simulink library "tqd"  (R2021b)
settings: Solver=VariableStepAuto  StartTime=0.0  StopTime=10.0  RelTol=1e-3
undefined symbols (not defined in the file or in its folder): ATQD_AccelLimitInRange_X_rpm, ATQD_AccelLimitInRange_Y_Nm, ATQD_AccelLimitOvrKi_X_Nm, ATQD_AccelLimitOvrKp_X_Nm, ATQD_BOSMapD_X_rpm, ATQD_BOSMapD_Y_pct, ATQD_BOSMapR_X_rpm, ATQD_BOSMapR_Y_pct, ATQD_HVBCurrSmooth_X_A, ATQD_LHMTqMapDLC_X_rpm, ATQD_LHMTqMapDLC_Y_pct, ATQD_LHMTqMapRLC_X_rpm, ATQD_LHMTqMapRLC_Y_pct, ATQD_NormalMapDLC_X_rpm, ATQD_NormalMapDLC_Y_pct, ATQD_NormalTqDecSR_X_rpm, ATQD_NormalTqDecSR_Y_Nm, ATQD_NormalTqIncSR_X_rpm, ATQD_NormalTqIncSR_Y_Nm, ATQD_OPDMapRLC_X_rpm, ATQD_OPDMapRLC_Y_pct, ATQD_RollRegTorReq_X_rpm, ATQD_RollRegTorReq_Y_enum, ATQD_VehSpdLimitInRange_X_rpm, ATQD_VehSpdLimitInRange_Y_Nm, ATQD_VehSpdLimitOvrKi_X_Nm, ATQD_VehSpdLimitOvrKp_X_Nm, EIGHT_INT, ENUM_BRAKEPEDAL_PRESSED, ENUM_BRAKEPEDAL_RELEASED, ENUM_COMBOKEY_DOWN, ENUM_COMBOKEY_M1, ENUM_COMBOKEY_M2, ENUM_COMBOKEY_NONE, ENUM_COMBOKEY_RKNEE, ENUM_COMBOKEY_STOPLV, ENUM_COMBOKEY_UP, ENUM_CP2VKNEEREQ_REQUEST, ENUM_CP2VNLVREQ_LEVEL1, ENUM_CP2VNLVREQ_LEVEL2, ENUM_CP2VNLVREQ_LOWER, ENUM_CP2VNLVREQ_STOPLV, ENUM_CP2VNLVREQ_UPPER, ENUM_CREEPIND_DISABLE, ENUM_CREEPIND_READY, ENUM_CREEPIND_RUNNING, ENUM_CREEPIND_WARNING, ENUM_DRIVELINERELEASE_RELEASE, ENUM_EBSTORQUERWQ_LIMIT, ENUM_EBSTORQUERWQ_TORQUE, ENUM_ECPVCUDRM_CONFORT, ENUM_ECPVCUDRM_ECO, ENUM_ECPVCUDRM_NORMAL, ENUM_ECPVCUDRM_NOTAVAILABLE, ENUM_EMTqModeDrvBrk_Accel, ENUM_EMTqModeDrvBrk_Brake, ENUM_EMTqModeDrvBrk_Coast, ENUM_ETC2ACTDRIVEDIR_BACKWARD, ENUM_ETC2ACTDRIVEDIR_FORWARD, ENUM_ETC2ACTDRIVEDIR_STILL ... (+341)
libraries: simulink x109, hcu_lib x67
(part 6 of 13)

== system tqd/TQD/Input_Convert/Function/Command Limitation ==
  note: Torque Command Lower Limit
  note: Torque Command Upper Limit
  BSCPIn_outputs : Inport
  BSignalConvert_outputs : Inport  Port=2
  VTQD_VehSpdTorLimit_Nm : Inport  Port=3
  VTQD_VehAcclTorLimit_Nm : Inport  Port=4
  Bus Selector : BusSelector  OutputSignals=VTQD_PTAvailMotTq_Nm,VTQD_EM1ReqTorqLimDriv_Nm,VTQD_EM1LimitCtrlDriv_flg,VTQD_TrqLimit_flg,VTQD_EM1ReqTorqLimBrk_Nm,VTQD_EM1LimitCtrlBrk_flg,VTQD_PTAvailGenTq_Nm
  Bus Selector1 : BusSelector  OutputSignals=VDMM_CAN1BUSOFF_flg
  Constant11 : Constant  Value=KTQD_PowerTrainTqLimtAtTargetShaft_Nm
  Constant16 : Constant  Value=KTQD_PowerTrainTqLimtAtTargetShaft_Nm
  Constant21 : Constant  Value=KTQD_PowerTrainTqLimtAtRegen_Nm
  Constant22 : Constant  Value=KTQD_DDMTrqLimitation_Nm
  Constant3 : Constant  Value=KTQD_CAN1BusOffTrqLimit_Nm
  LiuZgSwitch15 : Switch  Criteria=u2 ~= 0  Threshold=0.5
      settings: AttributesFormatString=<%<Criteria>>
  LiuZgSwitch16 : Switch  Criteria=u2 ~= 0  Threshold=0.5
      settings: AttributesFormatString=<%<Criteria>>
  MinMax3 : MinMax  Inputs=6  OutDataTypeStr=single
  MinMax4 : MinMax  Function=max  Inputs=3  OutDataTypeStr=single
  Switch4 : Switch  Criteria=u2 ~= 0
      settings: AttributesFormatString=%<Criteria>
  Switch5 : Switch  Criteria=u2 ~= 0
      settings: AttributesFormatString=%<Criteria>
  VTQD_TqCMDUpLim_Nm : Outport
  VTQD_TqCMDLowLim_Nm : Outport  Port=2
  wires:
  [VTQD_TqCMDLowLim_Nm] -> VTQD_TqCMDLowLim_Nm/1
  Bus Selector1/1 -> [VDMM_CAN1BUSOFF_flg]  "<VDMM_CAN1BUSOFF_flg>"
  BSCPIn_outputs/1 -> Bus Selector1/1
  Bus Selector/1 -> [VTQD_PTAvailMotTq_Nm]  "<VTQD_PTAvailMotTq_Nm>"
  BSignalConvert_outputs/1 -> Bus Selector/1
  VTQD_VehSpdTorLimit_Nm/1 -> [VTQD_VehSpdTorLimit_Nm]
  VTQD_VehAcclTorLimit_Nm/1 -> [VTQD_VehAcclTorLimit_Nm]
  [VTQD_EM1LimitCtrlDriv_flg] -> LiuZgSwitch15/2
  [VDMM_CAN1BUSOFF_flg] -> Switch4/2
  [VTQD_EM1ReqTorqLimDriv_Nm] -> LiuZgSwitch15/1
  Constant3/1 -> Switch4/1
  Constant11/1 -> Switch4/3
  [VTQD_TrqLimit_flg] -> Switch5/2
  Constant16/1 -> Switch5/3
  [VTQD_PTAvailMotTq_Nm] -> LiuZgSwitch15/3
  Constant22/1 -> Switch5/1
  Switch4/1 -> MinMax3/1
  [VTQD_PTAvailMotTq_Nm] -> MinMax3/2
  [VTQD_VehSpdTorLimit_Nm] -> MinMax3/3
  [VTQD_VehAcclTorLimit_Nm] -> MinMax3/4
  LiuZgSwitch15/1 -> MinMax3/5
  Switch5/1 -> MinMax3/6
  Bus Selector/2 -> [VTQD_EM1ReqTorqLimDriv_Nm]  "<VTQD_EM1ReqTorqLimDriv_Nm>"
  Bus Selector/3 -> [VTQD_EM1LimitCtrlDriv_flg]  "<VTQD_EM1LimitCtrlDriv_flg>"
  Bus Selector/4 -> [VTQD_TrqLimit_flg]  "<VTQD_TrqLimit_flg>"
  MinMax3/1 -> [VTQD_TqCMDUpLim_Nm]  "VTQD_TqCMDUpLim_Nm"
  [VTQD_EM1ReqTorqLimBrk_Nm] -> LiuZgSwitch16/1
  [VTQD_PTAvailGenTq_Nm] -> LiuZgSwitch16/3
  [VTQD_EM1LimitCtrlBrk_flg] -> LiuZgSwitch16/2
  Constant21/1 -> MinMax4/1
  LiuZgSwitch16/1 -> MinMax4/2
  [VTQD_PTAvailGenTq_Nm] -> MinMax4/3
  MinMax4/1 -> [VTQD_TqCMDLowLim_Nm]  "VTQD_TqCMDLowLim_Nm"
  Bus Selector/5 -> [VTQD_EM1ReqTorqLimBrk_Nm]  "<VTQD_EM1ReqTorqLimBrk_Nm>"
  Bus Selector/6 -> [VTQD_EM1LimitCtrlBrk_flg]  "<VTQD_EM1LimitCtrlBrk_flg>"
  Bus Selector/7 -> [VTQD_PTAvailGenTq_Nm]  "<VTQD_PTAvailGenTq_Nm>"
  [VTQD_TqCMDUpLim_Nm] -> VTQD_TqCMDUpLim_Nm/1

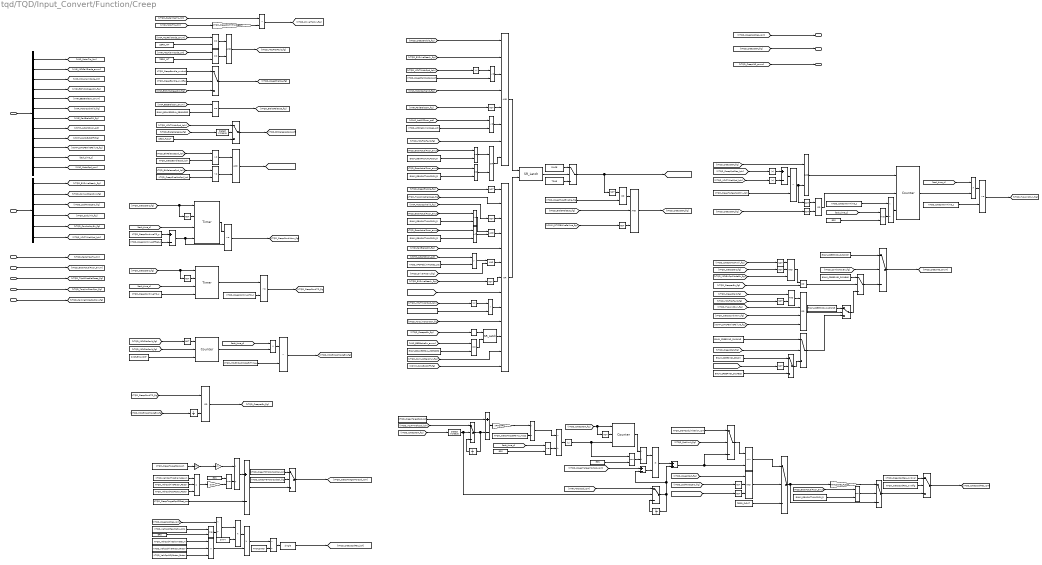
== system tqd/TQD/Input_Convert/Function/Creep ==
  note: TUpA Active Detection
  note: Creep SCP
  note: Creep Enable Judgment
  note: Creep Continue TimeOut
  note: MCU Error Condition
  note: Error Condition Judgment
  note: Unit Convert
  note: CmdSpeedCalculation
  note: Creep Indicate State
  BSCPIn_outputs : Inport
  BSignalConvert_outputs : Inport  Port=2
  VTQD_PedalMapTq_Nm : Inport  Port=3
  VTQD_GearActualPosn_enum : Inport  Port=4
  VTQD_TUpADisableCreep_flg : Inport  Port=5
  VTQD_TorqLimDoorOpn_flg : Inport  Port=6
  VTQD_ParkingProtectAction_flg : Inport  Port=7
  AND{,3,5..8} (6 alike) : Logic  AllPortsSameDT=off  OutDataTypeStr=boolean
  AND1 : Logic  Inputs=3  AllPortsSameDT=off  OutDataTypeStr=boolean
  AND2 : Logic  Inputs=3  AllPortsSameDT=off  OutDataTypeStr=boolean
  AND4 : Logic  Inputs=3  AllPortsSameDT=off  OutDataTypeStr=boolean
  Abs{,1,3..5} (5 alike) : Abs
  Add{,1,3..5} (5 alike) : Sum  Inputs=+-
  Add2 : Sum
  Bus Selector : BusSelector  OutputSignals=VTQD_EVDriveReady_flg,VTQD_ComLostZeroPwr_flg,VTQD_SpdForceZero_flg,VTQD_SpdLimit_flg,VTQD_ComboKeyEn_flg,VTQD_VCUTMVehSpd_kph
  Bus Selector1 : BusSelector  OutputSignals=VINP_MotorTrq_Nm,VINP_MCUFailGrade_enum,VINP_MCUAlarmCode_cnt,VINP_ECPVCUCreepSW_flg,VINP_EBSBrakeSw_enum,VINP_MotorSpdValid_flg,VINP_ParkBrakeSW_flg,VDHP_ActAPSPosn_pct,VDMM_CAN1BUSOFF_flg,VDMM_DTCPBWireFailure_flg,task_time_s,VINP_MotorSpd_rpm
  Constant : Constant  Value=ZERO_FLOAT  OutDataTypeStr=single
  Constant1 : Constant  Value=ENUM_BRAKEPEDAL_PRESSED
  Constant10 : Constant  Value=ENUM_GEARACTUALPOSN_R
  Constant11 : Constant  Value=ENUM_GEARACTUALPOSN_D
  Constant12 : Constant  Value=KTQD_APSPedLim4Creep_pct
  Constant13 : Constant  Value=KTQD_CreepContinueTO_s
  Constant14 : Constant  Value=KTQD_CreepTargetSpd_kph
  Constant15 : Constant  Value=KTQD_VehSpdTireDiameter_m
  Constant16 : Constant  Value=KTQD_VehSpdTireFactor_Factor
  Constant17 : Constant  Value=KTQD_CreepForedEnable_flg
  Constant18 : Constant  Value=KTQD_CreepTargetSpdOffset_rpm
  Constant19 : Constant  Value=KTQD_CreepTGMotorSpdCal_rpm
  Constant2 : Constant  Value=ENUM_GEARACTUALPOSN_R
  Constant20 : Constant  Value=FALSE
  Constant21 : Constant  Value=TRUE
  Constant22 : Constant  Value=ENUM_BRAKEPEDAL_RELEASED
  Constant23 : Constant  Value=ENUM_CREEPIND_DISABLE
  Constant24 : Constant  Value=KTQD_CreepTargetSpd_kph
  Constant25 : Constant  Value=KTQD_CreepTGMotorSpdCal_flg
  Constant26 : Constant  Value=ENUM_GEARACTUALPOSN_R
  Constant27 : Constant  Value=ENUM_GEARACTUALPOSN_D
  Constant28 : Constant  Value=KTQD_CreepTargetRamp_mps2
  Constant29 : Constant  Value=KTQD_CreepSpdReq_ovrdval
  Constant{3,9,31,55..56} (5 alike) : Constant  Value=EPS
  Constant30 : Constant  Value=KTQD_CreepSpdReq_ovrdflg
  Constant32 : Constant  Value=KTQD_CreepWarnTime_s
  Constant33 : Constant  Value=KTQD_CreepTartgerSpdDiv_kph
  Constant34 : Constant  Value=KTQD_VehSpdADJFactor_Factor
  Constant35 : Constant  Value=KTQD_VehSpdGearRatio_ratio
  Constant36 : Constant  Value=KTQD_VehSpdADJFactor_Factor
  Constant37 : Constant  Value=KTQD_CreepEanbleSpd_kph
  Constant38 : Constant  Value=KTQD_CreepWarnTime_s
  Constant39 : Constant  Value=ENUM_CREEPIND_WARNING
  Constant4 : Constant  Value=KTQD_CreepContinueTO_s
  Constant40 : Constant  Value=KTQD_CreepContinueOffset_s
  Constant41 : Constant  Value=KTQD_DDMSpdLimitation_rpm
  Constant42 : Constant  Value=SINGLEMAXCNT  OutDataTypeStr=single
  Constant43 : Constant  Value=KTQD_MCUEnSpdModeErrTime_s
  Constant44 : Constant  Value=KTQD_CreepDisableSpd_kph
  Constant45 : Constant  Value=ZERO_FLOAT
  Constant46 : Constant  Value=KTQD_VehSpdTireDiameter_m
  Constant47 : Constant  Value=KTQD_VehSpdTireFactor_Factor
  Constant48 : Constant  Value=ZERO_INT
  Constant49 : Constant  Value=SIXTY  OutDataTypeStr=single
  Constant5 : Constant  Value=KTQD_CreepEanble_ovrdval
  Constant50 : Constant  Value=ENUM_CREEPIND_RUNNING
  Constant51 : Constant  Value=ENUM_CREEPIND_READY
  Constant52 : Constant  Value=ENUM_CREEPIND_DISABLE
  Constant53 : Constant  Value=ENUM_CREEPIND_RUNNING
  Constant54 : Constant  Value=THOUSAND  OutDataTypeStr=single
  Constant58 : Constant  Value=KTQD_CreepForcedDisaSpd_kph
  Constant59 : Constant  Value=ZERO_INT
  Constant6 : Constant  Value=KTQD_CreepEanble_ovrdflg
  Constant60 : Constant  Value=KTQD_CreepContinueTO_s
  Constant7 : Constant  Value=KTQD_APSPedLim4Creep_pct
  Constant8 : Constant  Value=KTQD_CreepEanbleSpd_kph
  Counter : hcu_lib/Basic_Blocks/Counter
  Counter1 : hcu_lib/Basic_Blocks/Counter
  Counter4 : hcu_lib/Basic_Blocks/Counter
  Data Type Conversion : DataTypeConversion  OutDataTypeStr=single
  Detect Increase : simulink/Logic and Bit Operations/Detect Increase  vinit=boolean(0)  OutDataTypeStr=boolean
  Detect Increase1 : simulink/Logic and Bit Operations/Detect Increase  vinit=boolean(0)  OutDataTypeStr=boolean
  Divide{,1..4,6..7} (7 alike) : Product  Inputs=*/
  Divide5 : Product  Inputs=**
  Equal1 : RelationalOperator  Operator=<=  OutDataTypeStr=boolean  RndMeth=Simplest
  Equal{2,4..6,10..11,18} (7 alike) : RelationalOperator  Operator===  OutDataTypeStr=boolean  RndMeth=Simplest
  Equal14 : RelationalOperator  OutDataTypeStr=boolean  RndMeth=Simplest
  Equal15 : RelationalOperator  Operator=<=  OutDataTypeStr=boolean  RndMeth=Simplest
  Equal16 : RelationalOperator  Operator=>  OutDataTypeStr=boolean  RndMeth=Simplest
  Equal3 : RelationalOperator  Operator=<=  OutDataTypeStr=boolean  RndMeth=Simplest
  Equal7 : RelationalOperator  Operator=~=  OutDataTypeStr=boolean  RndMeth=Simplest
  Equal8 : RelationalOperator  Operator=~=  OutDataTypeStr=boolean  RndMeth=Simplest
  Equal9 : RelationalOperator  Operator=>  OutDataTypeStr=boolean  RndMeth=Simplest
  Gain1 : Gain  Gain=MINUSONE_FLOAT
  KDIP_VehSpdGearRatio_ratio : Gain  Gain=KTQD_VehSpdGearRatio_ratio
  KPH2MPS : Gain  Gain=KPH2MPS
  KTQD_CreepDisTMTorq_gain : Gain  Gain=KTQD_CreepDisTMTorq_gain
  Max{,1..4} (5 alike) : MinMax  Function=max  Inputs=2
  Memory : Memory  InitialCondition=boolean(0)  InheritSampleTime=on
      settings: AttributesFormatString=%<InitialCondition>
  Min : MinMax  Inputs=2
  Multiply2 : Gain  Gain=SIXTY  OutDataTypeStr=single
  NOT{,1..10,13..19} (18 alike) : Logic  Operator=NOT  AllPortsSameDT=off  OutDataTypeStr=boolean
  OR{,1,4..5,8} (5 alike) : Logic  Operator=OR  AllPortsSameDT=off  OutDataTypeStr=boolean
  OR2 : Logic  Inputs=8  AllPortsSameDT=off  OutDataTypeStr=boolean
  OR6 : Logic  Operator=OR  Inputs=13  AllPortsSameDT=off  OutDataTypeStr=boolean
  OR7 : Logic  Operator=OR  Inputs=4  AllPortsSameDT=off  OutDataTypeStr=boolean
  Product : Product  Inputs=3
  Product{1,3..5} (4 alike) : Product
  Product2 : Product  Inputs=3
  Relational Operator : RelationalOperator  Operator=>  OutDataTypeStr=boolean  RndMeth=Simplest
  Relational Operator1 : RelationalOperator  OutDataTypeStr=boolean  RndMeth=Simplest
  Relational Operator2 : RelationalOperator  OutDataTypeStr=boolean  RndMeth=Simplest
  Relational Operator3 : RelationalOperator  Operator=>  OutDataTypeStr=boolean  RndMeth=Simplest
  Relational Operator4 : RelationalOperator  Operator=>  OutDataTypeStr=boolean  RndMeth=Simplest
  Relational Operator7 : RelationalOperator  OutDataTypeStr=boolean  RndMeth=Simplest
  SR_Latch1 : hcu_lib/Basic_Blocks/SR_Latch
  SR_Latch2 : hcu_lib/Basic_Blocks/SR_Latch
  Switch{,1..14} (15 alike) : Switch  Criteria=u2 ~= 0
      settings: AttributesFormatString=%<Criteria>
  THOUSAND : Gain  Gain=THOUSAND
  Timer : hcu_lib/Basic_Blocks/Timer
  Timer2 : hcu_lib/Basic_Blocks/Timer
  Unit Delay : UnitDelay  InitialCondition=single(0)  SampleTime=-1  HasFrameUpgradeWarning=on
      settings: AttributesFormatString=%<InitialCondition>
  Unit Delay1 : UnitDelay  InitialCondition=single(0)  SampleTime=-1  HasFrameUpgradeWarning=on
      settings: AttributesFormatString=%<InitialCondition>
  Unit Delay2 : UnitDelay  InitialCondition=boolean(0)  SampleTime=-1  HasFrameUpgradeWarning=on
      settings: AttributesFormatString=%<InitialCondition>
  VTQD_CreepSpdReq_rpm : Outport
  VTQD_CreepStart_flg : Outport  Port=2
  VTQD_CreepIND_enum : Outport  Port=3
  wires:
  [VTQD_CreepSpdReq_rpm] -> VTQD_CreepSpdReq_rpm/1
  BSCPIn_outputs/1 -> Bus Selector1/1
  BSignalConvert_outputs/1 -> Bus Selector/1
  KTQD_CreepDisTMTorq_gain/1 -> Relational Operator3/2
  Relational Operator3/1 -> [VTQD_DriverTqOvr_flg]  "VTQD_DriverTqOvr_flg"
  [VTQD_PedalMapTq_Nm] -> Relational Operator3/1
  [VINP_MotorTrq_Nm] -> KTQD_CreepDisTMTorq_gain/1
  AND6/1 -> [VTQD_MCUFNoFault_flg]  "VTQD_MCUFNoFault_flg"
  Equal11/1 -> AND6/1
  Constant59/1 -> Equal18/2
  Equal18/1 -> AND6/2
  Constant48/1 -> Equal11/2
  [VINP_MCUFailGrade_enum] -> Equal11/1
  [VINP_MCUAlarmCode_cnt] -> Equal18/1
  Switch/1 -> [VTQD_CreepEnable_flg]  "VTQD_CreepEnable_flg"
  [VINP_ECPVCUCreepSW_flg] -> Switch/3
  Constant5/1 -> Switch/1
  Constant6/1 -> Switch/2
  Equal6/1 -> [VTQD_BrakeRelease_flg]  "VTQD_BrakeRelease_flg"
  [VINP_EBSBrakeSw_enum] -> Equal6/1
  Constant22/1 -> Equal6/2
  [VTQD_VCUTMVehSpd_kph] -> Switch8/1
  Constant45/1 -> Switch8/3
  [VTQD_BrakeRelease_flg] -> Detect Increase1/1
  Detect Increase1/1 -> Switch8/2
  Switch8/1 -> [VTQD_BrkReleaseSpd_kph]  "VTQD_BrkReleaseSpd_kph"
  Equal14/1 -> AND5/1
  Equal15/1 -> AND5/2
  AND5/1 -> [VTQD_VehBrkReleaseFail_flg]  "VTQD_VehBrkReleaseFail_flg"
  Constant44/1 -> Equal15/2
  [VTQD_BrkReleaseSpd_kph] -> Equal15/1
  [VTQD_BrkReleaseSpd_kph] -> Equal14/1
  Constant37/1 -> Equal14/2
  VTQD_PedalMapTq_Nm/1 -> [VTQD_PedalMapTq_Nm]
  [VDMM_DTCPBWireFailure_flg] -> NOT14/1
  Equal3/1 -> OR2/6
  [VTQD_EVDriveReady_flg] -> NOT9/1
  [VTQD_MCUFNoFault_flg] -> OR2/7
  [VTQD_DriverTqOvr_flg] -> AND8/2
  [VTQD_TorqLimDoorOpn_flg] -> OR6/10
  Memory/1 -> SR_Latch2/1
  Equal16/1 -> OR6/9
  Constant20/1 -> Switch2/1
  NOT6/1 -> OR6/3
  [VINP_ParkBrakeSW_flg] -> NOT1/1
  [VTQD_GearActualPosn_enum] -> Equal4/1
  Constant11/1 -> Equal5/2
  [VDHP_ActAPSPosn_pct] -> Equal9/1
  Equal5/1 -> OR1/2
  [VINP_MotorSpdValid_flg] -> NOT6/1
  SR_Latch2/1 -> OR6/11
  SR_Latch1/1 -> Switch2/2
  OR6/1 -> SR_Latch1/2
  Constant8/1 -> Equal1/2
  Equal10/1 -> SR_Latch2/2
  AND8/1 -> OR6/6
  Switch2/1 -> [VTQD_CreeperNotAvail_flg], NOT7/1  "VTQD_CreeperNotAvail_flg"
  Constant12/1 -> Equal9/2
  Constant7/1 -> Equal3/2
  NOT7/1 -> OR5/1
  [VTQD_CreeperErr_flg] -> Memory/1
  [VTQD_VehBrkReleaseFail_flg] -> OR6/8
  [VTQD_GearActualPosn_enum] -> Equal7/1
  [VDHP_ActAPSPosn_pct] -> Equal3/1
  [VTQD_CreepEnable_flg] -> OR2/1
  OR2/1 -> SR_Latch1/1
  NOT14/1 -> AND1/3
  [VTQD_ComLostZeroPwr_flg] -> OR6/12
  [VTQD_VCUTMVehSpd_kph] -> Abs5/1
  Constant58/1 -> Equal16/2
  Equal4/1 -> OR1/1
  Abs5/1 -> Equal16/1
  AND3/1 -> OR6/4
  [VTQD_BrakeRelease_flg] -> AND1/2
  [VTQD_TUpADisableCreep_flg] -> OR6/2
  [VTQD_CreepEnable_flg] -> NOT5/1
  NOT9/1 -> OR6/7
  Equal1/1 -> OR2/3
  Abs/1 -> Equal1/1
  Constant2/1 -> Equal7/2
  [VTQD_VCUTMVehSpd_kph] -> Abs/1
  Constant27/1 -> Equal8/2
  OR1/1 -> OR2/8
  [VTQD_GearActualPosn_enum] -> Equal5/1
  Equal8/1 -> AND3/2
  [VTQD_GearActualPosn_enum] -> Equal8/1
  Equal9/1 -> AND8/1
  [VDMM_CAN1BUSOFF_flg] -> OR6/13
  Constant10/1 -> Equal4/2
  [VINP_EBSBrakeSw_enum] -> Equal10/1
  [VINP_MotorSpdValid_flg] -> OR2/4
  Equal7/1 -> AND3/1
  NOT5/1 -> OR6/1
  NOT1/1 -> OR2/5
  AND1/1 -> [VTQD_CreepStart_flg]  "VTQD_CreepStart_flg"
  Constant17/1 -> OR5/2
  [VINP_ParkBrakeSW_flg] -> OR6/5
  [VTQD_EVDriveReady_flg] -> OR2/2
  OR5/1 -> AND1/1
  Constant21/1 -> Switch2/3
  Constant1/1 -> Equal10/2
  Bus Selector/1 -> [VTQD_EVDriveReady_flg]  "<VTQD_EVDriveReady_flg>"
  VTQD_GearActualPosn_enum/1 -> [VTQD_GearActualPosn_enum]
  VTQD_TUpADisableCreep_flg/1 -> [VTQD_TUpADisableCreep_flg]
  VTQD_TorqLimDoorOpn_flg/1 -> [VTQD_TorqLimDoorOpn_flg]
  Bus Selector/2 -> [VTQD_ComLostZeroPwr_flg]  "<VTQD_ComLostZeroPwr_flg>"
  NOT16/1 -> Timer2/2
  [VTQD_CreepStart_flg] -> Timer2/1, NOT16/1
  [VTQD_CreepStart_flg] -> Timer/1, NOT15/1
  [task_time_s] -> Timer2/3
  [task_time_s] -> Timer/3
  Timer2/1 -> Relational Operator2/1  "VTQD_CreepContinueTime_s"
  Constant4/1 -> Timer2/4
  Relational Operator2/1 -> [VTQD_CreepContiTO_flg]  "VTQD_CreepContiTO_flg"
  Constant40/1 -> Add/2
  Relational Operator7/1 -> [VTQD_CreepContiWarn_flg]  "VTQD_CreepContiWarn_flg"
  Constant13/1 -> Relational Operator2/2
  NOT15/1 -> Timer/2
  Add/1 -> Relational Operator7/2, Timer/4
  Timer/1 -> Relational Operator7/1
  Constant60/1 -> Add/1
  [task_time_s] -> Product5/1
  Constant43/1 -> Relational Operator4/2
  [VTQD_MCUFNoFault_flg] -> NOT13/1
  Relational Operator4/1 -> [VTQD_MCUEnSpdModeErr_flg]  "VTQD_MCUEnSpdModeErr_flg"
  Constant42/1 -> Counter4/3
  NOT13/1 -> Counter4/1
  [VTQD_MCUFNoFault_flg] -> Counter4/2
  Product5/1 -> Relational Operator4/1
  Counter4/1 -> Product5/2
  Unit Delay2/1 -> OR4/2
  OR4/1 -> [VTQD_CreeperErr_flg]  "VTQD_CreeperErr_flg"
  [VTQD_MCUEnSpdModeErr_flg] -> Unit Delay2/1
  [VTQD_CreepContiTO_flg] -> OR4/1
  Switch1/1 -> [VTQD_CreepTartgerMorSpd_rpm]  "VTQD_CreepTartgerMorSpd_rpm"
  Constant36/1 -> Product/3
  Constant14/1 -> THOUSAND/1
  Constant16/1 -> Product/2
  Constant19/1 -> Switch1/1
  Divide/1 -> Add1/1
  KDIP_VehSpdGearRatio_ratio/1 -> Divide/1
  Product/1 -> Multiply2/1
  THOUSAND/1 -> KDIP_VehSpdGearRatio_ratio/1
  Constant25/1 -> Switch1/2
  Add1/1 -> Switch1/3
  Constant18/1 -> Add1/2
  Constant15/1 -> Product/1
  [VTQD_CreepTartgerMorSpd_rpm] -> Add5/1
  NOT3/1 -> Counter/2
  NOT4/1 -> AND2/2
  [VTQD_ParkingProtectAction_flg] -> NOT19/1
  Switch3/1 -> Gain1/1, Switch9/3
  Abs1/1 -> Max2/1, Counter/3
  Switch4/1 -> Unit Delay/1, Add5/2, Add2/2
  KPH2MPS/1 -> Divide1/1
  [VTQD_SpdForceZero_flg] -> NOT4/1
  Unit Delay1/1 -> Switch6/3
  [VINP_MotorSpd_rpm] -> Switch4/1
  Constant26/1 -> Equal2/2
  Constant41/1 -> Switch5/1
  Product1/1 -> Add2/1
  [VTQD_CreepStart_flg] -> Counter/1, NOT3/1
  Constant29/1 -> Switch7/1
  Add5/1 -> Product1/2
  [VTQD_VCUTMVehSpd_kph] -> Switch6/1
  Gain1/1 -> Switch9/1
  Detect Increase/1 -> Switch4/2, Switch6/2
  Switch7/1 -> [VTQD_CreepSpdReq_rpm]  "VTQD_CreepSpdReq_rpm"
  Switch9/1 -> Switch7/3
  AND2/1 -> Switch3/2
  Switch6/1 -> Add3/2, Unit Delay1/1
  [VTQD_CreepStart_flg] -> AND2/1
  Add2/1 -> Switch5/3, Min/2
  Constant/1 -> Switch3/3
  Switch5/1 -> Min/1
  [VTQD_SpdLimit_flg] -> Switch5/2
  Counter/1 -> Divide3/1
  Min/1 -> Switch3/1  "VTQD_MinimizeSpdCMD_rpm"
  Add3/1 -> KPH2MPS/1
  Constant30/1 -> Switch7/2
  [VTQD_GearActualPosn_enum] -> Equal2/1
  Divide1/1 -> Divide2/1
  Equal2/1 -> Switch9/2
  Constant24/1 -> Add3/1
  Divide3/1 -> Product1/1
  Unit Delay/1 -> Switch4/3
  NOT19/1 -> AND2/3
  Divide2/1 -> Abs1/1
  Constant28/1 -> Divide1/2
  [VTQD_CreepStart_flg] -> Detect Increase/1
  Bus Selector/3 -> [VTQD_SpdForceZero_flg]  "<VTQD_SpdForceZero_flg>"
  VTQD_ParkingProtectAction_flg/1 -> [VTQD_ParkingProtectAction_flg]
  Bus Selector/4 -> [VTQD_SpdLimit_flg]  "<VTQD_SpdLimit_flg>"
  Switch14/1 -> Switch10/3
  [VTQD_CreepStart_flg] -> Switch10/2
  [VTQD_CreeperNotAvail_flg] -> NOT8/1
  Switch12/1 -> Switch13/3
  Switch11/1 -> Switch12/3
  Constant23/1 -> Switch12/1
  Constant51/1 -> Switch14/1
  Constant52/1 -> Switch14/3
  [VDMM_DTCPBWireFailure_flg] -> OR7/4
  Constant50/1 -> Switch10/1
  AND7/1 -> OR7/1
  NOT17/1 -> AND4/1
  NOT10/1 -> AND7/2
  OR7/1 -> Switch11/2
  Switch10/1 -> Switch11/3
  [VTQD_CreeperNotAvail_flg] -> NOT17/1
  [VTQD_ComboKeyEn_flg] -> Switch13/2
  Constant53/1 -> Switch13/1
  NOT18/1 -> AND4/2
  [VTQD_CreeperErr_flg] -> OR8/2
  AND4/1 -> OR8/1
  Switch13/1 -> [VTQD_CreepIND_enum]  "VTQD_CreepIND_enum"
  Constant39/1 -> Switch11/1
  [VTQD_MCUEnSpdModeErr_flg] -> AND4/3
  [VTQD_TUpAIndRun_flg] -> OR7/2
  [VTQD_CreepStart_flg] -> NOT18/1
  OR8/1 -> Switch12/2
  [VTQD_CreepContiWarn_flg] -> OR7/3
  NOT8/1 -> Switch14/2
  [VTQD_CreepStart_flg] -> AND7/1
  [VTQD_MCUFNoFault_flg] -> NOT10/1
  Bus Selector/5 -> [VTQD_ComboKeyEn_flg]  "<VTQD_ComboKeyEn_flg>"
  [VTQD_CreepStart_flg] -> VTQD_CreepStart_flg/1
  [VTQD_CreepIND_enum] -> VTQD_CreepIND_enum/1
  Max/1 -> Divide/2
  Multiply2/1 -> Max/2
  Constant3/1 -> Max/1
  Max1/1 -> Divide2/2
  [task_time_s] -> Max1/1
  Constant9/1 -> Max1/2
  Constant31/1 -> Max2/2
  Max2/1 -> Divide3/2
  [VTQD_CreepStart_flg] -> NOT2/1
  NOT2/1 -> OR/2
  NOT/1 -> OR/1
  AND/1 -> Counter1/1
  Divide4/1 -> Counter1/3
  Constant32/1 -> Divide4/1
  [VTQD_CreepStart_flg] -> AND/1
  Abs3/1 -> Add4/1
  [task_time_s] -> Product3/1
  Relational Operator1/1 -> [VTQD_TUpAIndRun_flg]  "VTQD_TUpAIndRun_flg"
  Add4/1 -> Relational Operator/1
  Constant33/1 -> Relational Operator/2
  [VTQD_CreepSpdReq_kph] -> Abs3/1
  Product3/1 -> Relational Operator1/1
  Relational Operator/1 -> AND/2, NOT/1
  [VTQD_VCUTMVehSpd_kph] -> Abs4/1
  Abs4/1 -> Add4/2
  Constant38/1 -> Relational Operator1/2
  OR/1 -> Counter1/2
  Counter1/1 -> Product3/2
  Data Type Conversion/1 -> [VTQD_CreepSpdReq_kph]  "VTQD_CreepSpdReq_kph"
  Constant34/1 -> Product2/3
  Divide7/1 -> Data Type Conversion/1
  Product4/1 -> Divide7/1
  Constant54/1 -> Divide7/2
  Product2/1 -> Product4/2
  Divide6/1 -> Divide5/1
  [VTQD_CreepSpdReq_rpm] -> Divide6/1
  Divide5/1 -> Product4/1
  Constant49/1 -> Divide5/2
  Constant46/1 -> Product2/1
  Constant47/1 -> Product2/2
  Max3/1 -> Divide6/2
  Constant35/1 -> Max3/1
  Constant55/1 -> Max3/2
  [task_time_s] -> Max4/1
  Max4/1 -> Divide4/2
  Constant56/1 -> Max4/2
  Bus Selector1/1 -> [VINP_MotorTrq_Nm]  "<VINP_MotorTrq_Nm>"
  Bus Selector1/2 -> [VINP_MCUFailGrade_enum]  "<VINP_MCUFailGrade_enum>"
  Bus Selector1/3 -> [VINP_MCUAlarmCode_cnt]  "<VINP_MCUAlarmCode_cnt>"
  Bus Selector1/4 -> [VINP_ECPVCUCreepSW_flg]  "<VINP_ECPVCUCreepSW_flg>"
  Bus Selector1/5 -> [VINP_EBSBrakeSw_enum]  "<VINP_EBSBrakeSw_enum>"
  Bus Selector1/6 -> [VINP_MotorSpdValid_flg]  "<VINP_MotorSpdValid_flg>"
  Bus Selector1/7 -> [VINP_ParkBrakeSW_flg]  "<VINP_ParkBrakeSW_flg>"
  Bus Selector1/8 -> [VDHP_ActAPSPosn_pct]  "<VDHP_ActAPSPosn_pct>"
  Bus Selector1/9 -> [VDMM_CAN1BUSOFF_flg]  "<VDMM_CAN1BUSOFF_flg>"
  Bus Selector1/10 -> [VDMM_DTCPBWireFailure_flg]  "<VDMM_DTCPBWireFailure_flg>"
  Bus Selector1/11 -> [task_time_s]  "<task_time_s>"
  Bus Selector1/12 -> [VINP_MotorSpd_rpm]  "<VINP_MotorSpd_rpm>"
  Bus Selector/6 -> [VTQD_VCUTMVehSpd_kph]  "<VTQD_VCUTMVehSpd_kph>"

== system tqd/TQD/Input_Convert/Function/Distribution Rate ==
  BSCPIn_outputs : Inport
  BSignalConvert_outputs : Inport  Port=2
  Constant1 : Constant  Value=KTQD_FrEDUSpRat_rat
  Constant2 : Constant  Value=KTQD_RrEDUSpRat_rat
  Terminator : Terminator
  Terminator1 : Terminator
  VTQD_FrEDUSpRat_rat : Outport
  VTQD_RrEDUSpRat_rat : Outport  Port=2
  wires:
  [VTQD_FrEDUSpRat_rat] -> VTQD_FrEDUSpRat_rat/1
  BSCPIn_outputs/1 -> Terminator/1
  BSignalConvert_outputs/1 -> Terminator1/1
  Constant1/1 -> [VTQD_FrEDUSpRat_rat]  "VTQD_FrEDUSpRat_rat"
  Constant2/1 -> [VTQD_RrEDUSpRat_rat]  "VTQD_RrEDUSpRat_rat"
  [VTQD_RrEDUSpRat_rat] -> VTQD_RrEDUSpRat_rat/1

== system tqd/TQD/Input_Convert/Function/Door Limit ==
  BSCPIn_outputs : Inport
  BSignalConvert_outputs : Inport  Port=2
  Bus Selector : BusSelector  OutputSignals=VTQD_DoorOpen_flg,VTQD_VCUVehSpd_kph
  Bus Selector1 : BusSelector  OutputSignals=VDSC_DoorSaftySW_flg,VDMM_DTCDoorStaError_flg,VDMM_DTCBCMDoorStaLostCom_flg
  Constant2 : Constant  Value=KTQD_SpeedThrDoorOpn_kph
  Logical Operator1 : Logic  Inputs=4  AllPortsSameDT=off  OutDataTypeStr=boolean
  Logical Operator2 : Logic  AllPortsSameDT=off  OutDataTypeStr=boolean
  NOT : Logic  Operator=NOT  AllPortsSameDT=off  OutDataTypeStr=boolean
  NOT1 : Logic  Operator=NOT  AllPortsSameDT=off  OutDataTypeStr=boolean
  Relational Operator : RelationalOperator  Operator=<  OutDataTypeStr=boolean  RndMeth=Simplest
  VTQD_TorqLimDoorOpn_flg : Outport
  wires:
  [VTQD_TorqLimDoorOpn_flg] -> VTQD_TorqLimDoorOpn_flg/1
  BSCPIn_outputs/1 -> Bus Selector1/1
  Bus Selector/1 -> [VTQD_DoorOpen_flg]  "<VTQD_DoorOpen_flg>"
  BSignalConvert_outputs/1 -> Bus Selector/1
  NOT/1 -> Logical Operator1/3
  Relational Operator/1 -> Logical Operator2/2
  NOT1/1 -> Logical Operator1/4
  Logical Operator2/1 -> Logical Operator1/1
  Constant2/1 -> Relational Operator/2
  Logical Operator1/1 -> [VTQD_TorqLimDoorOpn_flg]  "VTQD_TorqLimDoorOpn_flg"
  [VTQD_VCUVehSpd_kph] -> Relational Operator/1
  [VTQD_DoorOpen_flg] -> Logical Operator2/1
  [VDSC_DoorSaftySW_flg] -> Logical Operator1/2
  [VDMM_DTCDoorStaError_flg] -> NOT/1
  [VDMM_DTCBCMDoorStaLostCom_flg] -> NOT1/1
  Bus Selector/2 -> [VTQD_VCUVehSpd_kph]  "<VTQD_VCUVehSpd_kph>"
  Bus Selector1/3 -> [VDMM_DTCBCMDoorStaLostCom_flg]  "<VDMM_DTCBCMDoorStaLostCom_flg>"
  Bus Selector1/2 -> [VDMM_DTCDoorStaError_flg]  "<VDMM_DTCDoorStaError_flg>"
  Bus Selector1/1 -> [VDSC_DoorSaftySW_flg]  "<VDSC_DoorSaftySW_flg>"

== system tqd/TQD/Input_Convert/Function/MCU Control Mode ==
  BSCPIn_outputs : Inport
  BSignalConvert_outputs : Inport  Port=2
  VTQD_CreepStart_flg : Inport  Port=3
  VTQD_ParkingProtectAction_flg : Inport  Port=4
  AND : Logic  AllPortsSameDT=off  OutDataTypeStr=boolean
  Bus Selector : BusSelector  OutputSignals=VTQD_EVDriveReady_flg,VTQD_ForceDischarge_flg
  Bus Selector1 : BusSelector  OutputSignals=VPMM_SysPowerMode_enum,VPMM_VCUMCUCtrlMd_enum
  Constant : Constant  Value=ENUM_MCUCTRLMODE_NONE
  Constant1 : Constant  Value=ENUM_MCUCTRLMODE_TORQUE
  Constant2 : Constant  Value=ENUM_MCUCTRLMODE_SPEED
  Constant3 : Constant  Value=ENUM_PMMMODE_DRIVE
  Constant4 : Constant  Value=ENUM_MCUCTRLMODE_ACTDISCHRG
  Constant6 : Constant  Value=ENUM_MCUCTRLMODE_ACTDISCHRG
  Equal : RelationalOperator  Operator===  OutDataTypeStr=boolean  RndMeth=Simplest
  Equal1 : RelationalOperator  Operator===  OutDataTypeStr=boolean  RndMeth=Simplest
  OR : Logic  Operator=OR  AllPortsSameDT=off  OutDataTypeStr=boolean
  OR2 : Logic  Operator=OR  AllPortsSameDT=off  OutDataTypeStr=boolean
  Switch : Switch  Criteria=u2 ~= 0
      settings: AttributesFormatString=%<Criteria>
  Switch1 : Switch  Criteria=u2 ~= 0
      settings: AttributesFormatString=%<Criteria>
  Switch2 : Switch  Criteria=u2 ~= 0
      settings: AttributesFormatString=%<Criteria>
  VTQD_VCUMCUCtrlMdTQD_enum : Outport
  wires:
  BSignalConvert_outputs/1 -> Bus Selector/1
  Bus Selector/1 -> [VTQD_EVDriveReady_flg]  "<VTQD_EVDriveReady_flg>"
  BSCPIn_outputs/1 -> Bus Selector1/1
  Bus Selector1/1 -> [VPMM_SysPowerMode_enum]  "<VPMM_SysPowerMode_enum>"
  Bus Selector1/2 -> [VPMM_VCUMCUCtrlMd_enum]  "<VPMM_VCUMCUCtrlMd_enum>"
  [VTQD_ForceDischarge_flg] -> AND/1
  Switch/1 -> Switch1/3
  [VTQD_EVDriveReady_flg] -> Switch/2
  [VTQD_ParkingProtectAction_flg] -> OR2/2
  Switch1/1 -> Switch2/3
  Constant4/1 -> Equal/2
  Constant2/1 -> Switch1/1
  Constant1/1 -> Switch/1
  OR2/1 -> Switch1/2
  [VTQD_CreepStart_flg] -> OR2/1
  Constant3/1 -> Equal1/2
  Constant6/1 -> Switch2/1
  AND/1 -> OR/1
  OR/1 -> Switch2/2
  Equal1/1 -> AND/2
  Switch2/1 -> [VTQD_VCUMCUCtrlMdTQD_enum]  "VTQD_VCUMCUCtrlMdTQD_enum"
  Equal/1 -> OR/2
  Constant/1 -> Switch/3
  [VTQD_VCUMCUCtrlMdTQD_enum] -> VTQD_VCUMCUCtrlMdTQD_enum/1
  Bus Selector/2 -> [VTQD_ForceDischarge_flg]  "<VTQD_ForceDischarge_flg>"
  VTQD_ParkingProtectAction_flg/1 -> [VTQD_ParkingProtectAction_flg]
  VTQD_CreepStart_flg/1 -> [VTQD_CreepStart_flg]
  [VPMM_VCUMCUCtrlMd_enum] -> Equal/1
  [VPMM_SysPowerMode_enum] -> Equal1/1

== system tqd/TQD/Input_Convert/Function/Parking Protection ==
  BSCPIn_outputs : Inport
  BSignalConvert_outputs : Inport  Port=2
  VTQD_GearActualPosn_enum : Inport  Port=3
  AND : Logic  Inputs=3  AllPortsSameDT=off  OutDataTypeStr=boolean
  AND1 : Logic  Inputs=3  AllPortsSameDT=off  OutDataTypeStr=boolean
  AND2 : Logic  AllPortsSameDT=off  OutDataTypeStr=boolean
  AND6 : Logic  Inputs=6  AllPortsSameDT=off  OutDataTypeStr=boolean
  AND7 : Logic  Inputs=4  AllPortsSameDT=off  OutDataTypeStr=boolean
  Bus Selector : BusSelector  OutputSignals=VTQD_LVchrgSvrMode_flg,VTQD_DoorOpen_flg,VTQD_AccelPedalDepressed_flg,VTQD_VCUVehSpd_kph
  Bus Selector1 : BusSelector  OutputSignals=VINP_MotorSpd_rpm,VDSC_DoorSaftySW_flg,VDMM_DTCDoorStaError_flg,VDMM_DTCBCMDoorStaLostCom_flg,VINP_SeatBeltSta_flg,VINP_ParkBrakeSW_flg,VINP_EBSBrakeSw_enum,task_time_s,VPMM_SysPowerMode_enum
  Constant : Constant  Value=KTQD_noPBDetectSpd_kph
  Constant1 : Constant  Value=ENUM_BRAKEPEDAL_RELEASED
  Constant11 : Constant  Value=KTQD_ParkSafeDoorOpenSW_ovrdflg
  Constant12 : Constant  Value=KTQD_ParkSafeDoorOpenSW_ovrdval
  Constant16 : Constant  Value=KTQD_ParkSafeSeatBeltSW_ovrdflg
  Constant17 : Constant  Value=KTQD_ParkSafeSeatBeltSW_ovrdval
  Constant2 : Constant  Value=KTQD_noPBWarnPreActBuzzer_s
  Constant26 : Constant  Value=ENUM_GEARACTUALPOSN_D
  Constant3 : Constant  Value=KTQD_noPBStillSpd_kph
  Constant39 : Constant  Value=ENUM_GEARACTUALPOSN_R
  Constant4 : Constant  Value=KTQD_noPBDetectTMSpd_rpm
  Constant40 : Constant  Value=ENUM_GEARACTUALPOSN_N
  Constant5 : Constant  Value=KTQD_noPBStillTMSpd_rpm
  Constant6 : Constant  Value=FALSE
  Constant7 : Constant  Value=ENUM_BRAKEPEDAL_PRESSED
  Constant8 : Constant  Value=ENUM_PMMMODE_AFTERRUN
  Constant9 : Constant  Value=ENUM_PMMMODE_STANDBY
  Equal{,2..4,9..11} (7 alike) : RelationalOperator  Operator===  OutDataTypeStr=boolean  RndMeth=Simplest
  NOT{,1..6} (7 alike) : Logic  Operator=NOT  AllPortsSameDT=off  OutDataTypeStr=boolean
  OR : Logic  Operator=OR  Inputs=3  AllPortsSameDT=off  OutDataTypeStr=boolean
  OR1 : Logic  Operator=OR  AllPortsSameDT=off  OutDataTypeStr=boolean
  OR2 : Logic  Operator=OR  AllPortsSameDT=off  OutDataTypeStr=boolean
  OR4 : Logic  Operator=OR  AllPortsSameDT=off  OutDataTypeStr=boolean
  Relational Operator : RelationalOperator  OutDataTypeStr=boolean  RndMeth=Simplest
  Relational Operator{1..2,6..7} (4 alike) : RelationalOperator  Operator=<=  OutDataTypeStr=boolean  RndMeth=Simplest
  SR_Latch : hcu_lib/Basic_Blocks/SR_Latch
  Switch : Switch  Criteria=u2 ~= 0
      settings: AttributesFormatString=%<Criteria>
  Switch1 : Switch  Criteria=u2 ~= 0
      settings: AttributesFormatString=%<Criteria>
  Switch2 : Switch  Criteria=u2 ~= 0
      settings: AttributesFormatString=%<Criteria>
  Timer : hcu_lib/Basic_Blocks/Timer
  VTQD_ParkingProtectWarning_flg : Outport
  VTQD_ParkingProtectAction_flg : Outport  Port=2
  wires:
  [VTQD_ParkingProtectWarning_flg] -> VTQD_ParkingProtectWarning_flg/1
  BSCPIn_outputs/1 -> Bus Selector1/1
  Bus Selector/1 -> [VTQD_LVchrgSvrMode_flg]  "<VTQD_LVchrgSvrMode_flg>"
  BSignalConvert_outputs/1 -> Bus Selector/1
  NOT3/1 -> AND6/6
  AND/1 -> [VTQD_ParkingProtectAction_flg]  "VTQD_ParkingProtectAction_flg"
  SR_Latch/1 -> [VTQD_ParkingProtectWarning_flg], AND/1  "VTQD_ParkingProtectWarning_flg"
  Constant12/1 -> Switch1/3
  Constant17/1 -> Switch2/3
  [VDMM_DTCBCMDoorStaLostCom_flg] -> NOT3/1
  OR2/1 -> AND7/4
  Relational Operator6/1 -> AND6/1
  Relational Operator1/1 -> AND/2
  OR/1 -> SR_Latch/2  "VTQD_ParkingProtectRelease_flg"
  AND1/1 -> OR/2
  AND7/1 -> NOT/1, Timer/1  "VTQD_ParkingProtectWarnCrit_flg"
  Constant40/1 -> Equal11/2
  NOT1/1 -> Switch2/1
  Constant39/1 -> Equal10/2
  Constant26/1 -> Equal9/2
  [VTQD_GearActualPosn_enum] -> Equal10/1
  [VTQD_GearActualPosn_enum] -> Equal9/1
  Equal11/1 -> AND2/2
  [VINP_SeatBeltSta_flg] -> NOT1/1
  NOT6/1 -> AND1/2
  Constant16/1 -> Switch2/2
  Equal4/1 -> OR1/2
  [VINP_MotorSpd_rpm] -> Relational Operator2/1
  [VINP_ParkBrakeSW_flg] -> NOT5/1
  Equal9/1 -> OR4/1
  [VTQD_LVchrgSvrMode_flg] -> NOT4/1
  [task_time_s] -> Timer/3
  [VTQD_DoorOpen_flg] -> NOT6/1
  Constant2/1 -> Relational Operator/2, Timer/4
  Switch2/1 -> AND2/1
  [VINP_EBSBrakeSw_enum] -> Equal/1
  NOT2/1 -> AND6/5
  [VINP_MotorSpd_rpm] -> Relational Operator7/1
  Switch/1 -> OR/3
  Relational Operator7/1 -> AND6/2
  NOT/1 -> Timer/2
  Relational Operator2/1 -> AND/3
  Equal3/1 -> OR1/1
  AND2/1 -> OR2/2  "VTQD_NoPBSeatBelt_flg"
  Constant3/1 -> Relational Operator1/2
  Constant5/1 -> Relational Operator2/2
  Timer/1 -> Relational Operator/1
  NOT4/1 -> AND6/3
  [VDSC_DoorSaftySW_flg] -> AND6/4
  Constant8/1 -> Equal3/2
  [VTQD_VCUVehSpd_kph] -> Relational Operator1/1
  Equal/1 -> AND7/3
  [VTQD_AccelPedalDepressed_flg] -> AND1/1
  [VTQD_DoorOpen_flg] -> Switch1/1
  Constant1/1 -> Equal/2
  [VDMM_DTCDoorStaError_flg] -> NOT2/1
  [VINP_EBSBrakeSw_enum] -> Equal2/1
  Switch1/1 -> OR2/1  "VTQD_NoPBDoorOpen_flg"
  [VPMM_SysPowerMode_enum] -> Equal4/1
  [VTQD_VCUVehSpd_kph] -> Relational Operator6/1
  [VINP_ParkBrakeSW_flg] -> OR/1
  Equal2/1 -> Switch/3
  AND6/1 -> AND7/1  "VTQD_ParkingProtectWarnWind_flg"
  OR1/1 -> Switch/2
  Constant11/1 -> Switch1/2
  Equal10/1 -> OR4/2
  NOT5/1 -> AND7/2
  Constant9/1 -> Equal4/2
  Constant6/1 -> Switch/1
  Constant/1 -> Relational Operator6/2
  OR4/1 -> AND1/3
  [VPMM_SysPowerMode_enum] -> Equal3/1
  Constant7/1 -> Equal2/2
  Relational Operator/1 -> SR_Latch/1
  [VTQD_GearActualPosn_enum] -> Equal11/1
  Constant4/1 -> Relational Operator7/2
  Bus Selector/2 -> [VTQD_DoorOpen_flg]  "<VTQD_DoorOpen_flg>"
  VTQD_GearActualPosn_enum/1 -> [VTQD_GearActualPosn_enum]
  Bus Selector/3 -> [VTQD_AccelPedalDepressed_flg]  "<VTQD_AccelPedalDepressed_flg>"
  [VTQD_ParkingProtectAction_flg] -> VTQD_ParkingProtectAction_flg/1
  Bus Selector1/1 -> [VINP_MotorSpd_rpm]  "<VINP_MotorSpd_rpm>"
  Bus Selector1/2 -> [VDSC_DoorSaftySW_flg]  "<VDSC_DoorSaftySW_flg>"
  Bus Selector1/3 -> [VDMM_DTCDoorStaError_flg]  "<VDMM_DTCDoorStaError_flg>"
  Bus Selector1/4 -> [VDMM_DTCBCMDoorStaLostCom_flg]  "<VDMM_DTCBCMDoorStaLostCom_flg>"
  Bus Selector1/5 -> [VINP_SeatBeltSta_flg]  "<VINP_SeatBeltSta_flg>"
  Bus Selector1/6 -> [VINP_ParkBrakeSW_flg]  "<VINP_ParkBrakeSW_flg>"
  Bus Selector1/7 -> [VINP_EBSBrakeSw_enum]  "<VINP_EBSBrakeSw_enum>"
  Bus Selector1/8 -> [task_time_s]  "<task_time_s>"
  Bus Selector1/9 -> [VPMM_SysPowerMode_enum]  "<VPMM_SysPowerMode_enum>"
  Bus Selector/4 -> [VTQD_VCUVehSpd_kph]  "<VTQD_VCUVehSpd_kph>"

== system tqd/TQD/Input_Convert/Function/Pedal Torque ==
  note: Torque Command Determination
  note: Pedal Torque Map
  BSCPIn_outputs : Inport
  BSignalConvert_outputs : Inport  Port=2
  VTQD_GearActualPosn_enum : Inport  Port=3
  Bus Selector : BusSelector  OutputSignals=VTQD_TqTargetShaftSpd_rpm,VTQD_ActDriveMode_enum
  Bus Selector1 : BusSelector  OutputSignals=VDHP_ActAPSPosn_pct
  Constant : Constant  Value=FALSE
  MTQD_ConfortTqMapDLC_Z_Nm : Lookup_n-D  BreakpointsForDimension1=ATQD_NormalMapDLC_Y_pct  BreakpointsForDimension2=ATQD_NormalMapDLC_X_rpm  Table=MTQD_ConfortTqMapDLC_Z_Nm  InternalRulePriority=Speed  RndMeth=Simplest  InputSameDT=on
      settings: InputPortMap=u0,u1
  MTQD_ECOTqMapDLC_Z_Nm : Lookup_n-D  BreakpointsForDimension1=ATQD_NormalMapDLC_Y_pct  BreakpointsForDimension2=ATQD_NormalMapDLC_X_rpm  Table=MTQD_ECOTqMapDLC_Z_Nm  InternalRulePriority=Speed  RndMeth=Simplest  InputSameDT=on
      settings: InputPortMap=u0,u1
  MTQD_LHMTqMapDLC_Z_Nm : Lookup_n-D  BreakpointsForDimension1=ATQD_LHMTqMapDLC_Y_pct  BreakpointsForDimension2=ATQD_LHMTqMapDLC_X_rpm  Table=MTQD_LHMTqMapDLC_Z_Nm  InternalRulePriority=Speed  RndMeth=Simplest  InputSameDT=on
      settings: InputPortMap=u0,u1
  MTQD_LHMTqMapRLC_Z_Nm : Lookup_n-D  BreakpointsForDimension1=ATQD_LHMTqMapRLC_Y_pct  BreakpointsForDimension2=ATQD_LHMTqMapRLC_X_rpm  Table=MTQD_LHMTqMapRLC_Z_Nm  InternalRulePriority=Speed  RndMeth=Simplest  InputSameDT=on
      settings: InputPortMap=u0,u1
  MTQD_NormalMapDLC_Z_Nm : Lookup_n-D  BreakpointsForDimension1=ATQD_NormalMapDLC_Y_pct  BreakpointsForDimension2=ATQD_NormalMapDLC_X_rpm  Table=MTQD_NormalMapDLC_Z_Nm  InternalRulePriority=Speed  RndMeth=Simplest  InputSameDT=on
      settings: InputPortMap=u0,u1
  MTQD_OPDMapRLC_Z_Nm : Lookup_n-D  BreakpointsForDimension1=ATQD_OPDMapRLC_Y_pct  BreakpointsForDimension2=ATQD_OPDMapRLC_X_rpm  Table=MTQD_OPDMapRLC_Z_Nm  InternalRulePriority=Speed  RndMeth=Simplest  InputSameDT=on
      settings: InputPortMap=u0,u1
  Torque Command Determination : Stateflow chart  TreatAsAtomicUnit=on
  VTQD_PedalMapTq_Nm : Outport
  wires:
  BSignalConvert_outputs/1 -> Bus Selector/1
  Bus Selector/1 -> [VTQD_TqTargetShaftSpd_rpm]  "<VTQD_TqTargetShaftSpd_rpm>"
  BSCPIn_outputs/1 -> Bus Selector1/1
  [VTQD_PedalMapTq_Nm] -> VTQD_PedalMapTq_Nm/1
  [VTQD_TqTargetShaftSpd_rpm] -> MTQD_LHMTqMapDLC_Z_Nm/2
  [VDHP_ActAPSPosn_pct] -> MTQD_NormalMapDLC_Z_Nm/1
  [VDHP_ActAPSPosn_pct] -> MTQD_LHMTqMapDLC_Z_Nm/1
  [VDHP_ActAPSPosn_pct] -> MTQD_ECOTqMapDLC_Z_Nm/1
  MTQD_ECOTqMapDLC_Z_Nm/1 -> [VTQD_ECOTqMapD_Nm]  "VTQD_ECOTqMapD_Nm"
  [VTQD_TqTargetShaftSpd_rpm] -> MTQD_NormalMapDLC_Z_Nm/2
  [VTQD_TqTargetShaftSpd_rpm] -> MTQD_ECOTqMapDLC_Z_Nm/2
  [VTQD_TqTargetShaftSpd_rpm] -> MTQD_ConfortTqMapDLC_Z_Nm/2
  [VDHP_ActAPSPosn_pct] -> MTQD_ConfortTqMapDLC_Z_Nm/1
  MTQD_LHMTqMapDLC_Z_Nm/1 -> [VTQD_LHMTqMapD_Nm]  "VTQD_LHMTqMapD_Nm"
  MTQD_NormalMapDLC_Z_Nm/1 -> [VTQD_NormalTqMapD_Nm]  "VTQD_NormalTqMapD_Nm"
  MTQD_ConfortTqMapDLC_Z_Nm/1 -> [VTQD_ConfortTqMapD_Nm]  "VTQD_ConfortTqMapD_Nm"
  [VDHP_ActAPSPosn_pct] -> MTQD_OPDMapRLC_Z_Nm/1
  [VTQD_TqTargetShaftSpd_rpm] -> MTQD_OPDMapRLC_Z_Nm/2
  [VTQD_TqTargetShaftSpd_rpm] -> MTQD_LHMTqMapRLC_Z_Nm/2
  [VDHP_ActAPSPosn_pct] -> MTQD_LHMTqMapRLC_Z_Nm/1
  MTQD_OPDMapRLC_Z_Nm/1 -> [VTQD_OPDMapRLC_Nm]  "VTQD_OPDMapRLC_Nm"
  MTQD_LHMTqMapRLC_Z_Nm/1 -> [VTQD_LHMTqMapRLC_Nm]  "VTQD_LHMTqMapRLC_Nm"
  Bus Selector1/1 -> [VDHP_ActAPSPosn_pct]  "<VDHP_ActAPSPosn_pct>"
  [VTQD_GearActualPosn_enum] -> Torque Command Determination/1(VTQD_GearActualPosn_enum)
  [VTQD_ActDriveMode_enum] -> Torque Command Determination/2(VTQD_ActDriveMode_enum)
  Bus Selector/2 -> [VTQD_ActDriveMode_enum]  "<VTQD_ActDriveMode_enum>"
  VTQD_GearActualPosn_enum/1 -> [VTQD_GearActualPosn_enum]
  Constant/1 -> Torque Command Determination/3(VDHP_LHMRestrictDrivePwr_flg)  "VDHP_LHMRestrictDrivePwr_flg"
  [VTQD_NormalTqMapD_Nm] -> Torque Command Determination/4(VTQD_NormalTqMapD_Nm)
  [VTQD_ECOTqMapD_Nm] -> Torque Command Determination/5(VTQD_ECOTqMapD_Nm)
  [VTQD_ConfortTqMapD_Nm] -> Torque Command Determination/6(VTQD_ConfortTqMapD_Nm)
  [VTQD_OPDMapRLC_Nm] -> Torque Command Determination/7(VTQD_OPDMapRLC_Nm)
  [VTQD_LHMTqMapRLC_Nm] -> Torque Command Determination/8(VTQD_LHMTqMapRLC_Nm)
  [VTQD_LHMTqMapD_Nm] -> Torque Command Determination/9(VTQD_LHMTqMapD_Nm)
  Torque Command Determination/1(VTQD_PedalMapTq_Nm) -> [VTQD_PedalMapTq_Nm]

== system tqd/TQD/Input_Convert/Function/Ramp Limitation ==
  BSCPIn_outputs : Inport
  BSignalConvert_outputs : Inport  Port=2
  Constant1 : Constant  Value=KTQD_FinalTrqUpLim_Nm
  Constant2 : Constant  Value=KTQD_FinalTrqLowLim_Nm
  Terminator : Terminator
  Terminator1 : Terminator
  VTQD_FinalTrqUpLim_Nm : Outport
  VTQD_FinalTrqLowLim_Nm : Outport  Port=2
  wires:
  [VTQD_FinalTrqLowLim_Nm] -> VTQD_FinalTrqLowLim_Nm/1
  Constant2/1 -> [VTQD_FinalTrqLowLim_Nm]  "VTQD_FinalTrqLowLim_Nm"
  Constant1/1 -> [VTQD_FinalTrqUpLim_Nm]  "VTQD_FinalTrqUpLim_Nm"
  BSignalConvert_outputs/1 -> Terminator1/1
  BSCPIn_outputs/1 -> Terminator/1
  [VTQD_FinalTrqUpLim_Nm] -> VTQD_FinalTrqUpLim_Nm/1

== system tqd/TQD/Input_Convert/Function/Ramp Parameter ==
  note: Parameter Determination
  note: Torque Positive/Negative Change Judgment
  note: Ramp Map
  BSCPIn_outputs : Inport
  BSignalConvert_outputs : Inport  Port=2
  BMain_outputs : Inport  Port=3
  Abs{,1,3..6} (6 alike) : Abs
  Bus Selector : BusSelector  OutputSignals=VTQD_TMSpd_rpm,VTQD_TqSource_enum,VTQD_ActDriveMode_enum
  Bus Selector1 : BusSelector  OutputSignals=task_time_s
  Bus Selector2 : BusSelector  OutputSignals=VTQD_RrRampTq_Nm,VTQD_AfterAvailableTqDemRr_Nm
  Constant1 : Constant  Value=ZERO_FLOAT
  Constant2 : Constant  Value=ZERO_FLOAT
  Constant3 : Constant  Value=ZERO_FLOAT
  Constant4 : Constant  Value=MAX16BITCNT
  Counter : hcu_lib/Basic_Blocks/Counter
      settings: SourceProductName=HCU Relative Block Library
  Detect Decrease : simulink/Logic and Bit Operations/Detect Decrease  vinit=boolean(0)  OutDataTypeStr=boolean
  KTQD_POSNEGSWSMOTIME_s : Constant  Value=KTQD_POSNEGSWSMOTIME_s  OutDataTypeStr=single
  MTQD_ConfortTqDecSR_Z_Nm : Lookup_n-D  BreakpointsForDimension1=ATQD_NormalTqDecSR_Y_Nm  BreakpointsForDimension2=ATQD_NormalTqDecSR_X_rpm  Table=MTQD_ConfortTqDecSR_Z_Nm  InternalRulePriority=Speed  RndMeth=Simplest  InputSameDT=on
      settings: InputPortMap=u0,u1
  MTQD_ConfortTqIncSR_Z_Nm : Lookup_n-D  BreakpointsForDimension1=ATQD_NormalTqIncSR_Y_Nm  BreakpointsForDimension2=ATQD_NormalTqIncSR_X_rpm  Table=MTQD_ConfortTqIncSR_Z_Nm  InternalRulePriority=Speed  RndMeth=Simplest  InputSameDT=on
      settings: InputPortMap=u0,u1
  MTQD_ECOTqDecSR_Z_Nm : Lookup_n-D  BreakpointsForDimension1=ATQD_NormalTqDecSR_Y_Nm  BreakpointsForDimension2=ATQD_NormalTqDecSR_X_rpm  Table=MTQD_ECOTqDecSR_Z_Nm  InternalRulePriority=Speed  RndMeth=Simplest  InputSameDT=on
      settings: InputPortMap=u0,u1
  MTQD_ECOTqIncSR_Z_Nm : Lookup_n-D  BreakpointsForDimension1=ATQD_NormalTqIncSR_Y_Nm  BreakpointsForDimension2=ATQD_NormalTqIncSR_X_rpm  Table=MTQD_ECOTqIncSR_Z_Nm  InternalRulePriority=Speed  RndMeth=Simplest  InputSameDT=on
      settings: InputPortMap=u0,u1
  MTQD_NormalTqDecSR_Z_Nm : Lookup_n-D  BreakpointsForDimension1=ATQD_NormalTqDecSR_Y_Nm  BreakpointsForDimension2=ATQD_NormalTqDecSR_X_rpm  Table=MTQD_NormalTqDecSR_Z_Nm  InternalRulePriority=Speed  RndMeth=Simplest  InputSameDT=on
      settings: InputPortMap=u0,u1
  MTQD_NormalTqIncSR_Z_Nm : Lookup_n-D  BreakpointsForDimension1=ATQD_NormalTqIncSR_Y_Nm  BreakpointsForDimension2=ATQD_NormalTqIncSR_X_rpm  Table=MTQD_NormalTqIncSR_Z_Nm  InternalRulePriority=Speed  RndMeth=Simplest  InputSameDT=on
      settings: InputPortMap=u0,u1
  OR : Logic  Operator=OR  AllPortsSameDT=off  OutDataTypeStr=boolean
  Product : Product
  Ramp Parameter Determination : Stateflow chart  TreatAsAtomicUnit=on
  Relational Operator : RelationalOperator  Operator=>  OutDataTypeStr=boolean  RndMeth=Simplest
  Relational Operator1 : RelationalOperator  Operator=<  OutDataTypeStr=boolean  RndMeth=Simplest
  Relational Operator2 : RelationalOperator  Operator=>  OutDataTypeStr=boolean  RndMeth=Simplest
  Relational Operator3 : RelationalOperator  Operator=>  OutDataTypeStr=boolean  RndMeth=Simplest
  SR_Latch : hcu_lib/Basic_Blocks/SR_Latch
      settings: SourceProductName=HCU Relative Block Library
  SR_Latch1 : hcu_lib/Basic_Blocks/SR_Latch
      settings: SourceProductName=HCU Relative Block Library
  Saturation{,1,4,6,8,10} (6 alike) : Saturate  UpperLimit=3300  LowerLimit=0
      settings: AttributesFormatString=|
      | UpperLimit:%<UpperLimit>
      | LowerLimit:%<LowerLimit>
  Saturation{2..3,5,7,9,11} (6 alike) : Saturate  UpperLimit=3500  LowerLimit=-3500
      settings: AttributesFormatString=|
      | UpperLimit:%<UpperLimit>
      | LowerLimit:%<LowerLimit>
  Unit Delay : UnitDelay  InitialCondition=boolean(0)  SampleTime=-1  HasFrameUpgradeWarning=on
      settings: AttributesFormatString=%<InitialCondition>
  VTQD_RampTs_c : Outport
  VTQD_RampTqIncSR_Nm : Outport  Port=2
  VTQD_RampTqDecSR_Nm : Outport  Port=3
  wires:
  [VTQD_RampTs_c] -> VTQD_RampTs_c/1
  BSCPIn_outputs/1 -> Bus Selector1/1
  Bus Selector/1 -> [VTQD_TMSpd_rpm]  "<VTQD_TMSpd_rpm>"
  BSignalConvert_outputs/1 -> Bus Selector/1
  MTQD_ECOTqIncSR_Z_Nm/1 -> [VTQD_ECOTqIncSR_Nm]  "VTQD_ECOTqIncSR_Nm"
  [VTQD_TMSpd_rpm] -> Saturation11/1
  [VTQD_RrRampTq_Nm] -> Abs6/1
  [VTQD_TMSpd_rpm] -> Saturation9/1
  [VTQD_RrRampTq_Nm] -> Abs3/1
  [VTQD_TMSpd_rpm] -> Saturation7/1
  Abs4/1 -> Saturation6/1
  Abs/1 -> Saturation/1
  MTQD_NormalTqIncSR_Z_Nm/1 -> [VTQD_NormalTqIncSR_Nm]  "VTQD_NormalTqIncSR_Nm"
  Saturation2/1 -> MTQD_NormalTqIncSR_Z_Nm/2
  Abs3/1 -> Saturation4/1
  Saturation10/1 -> MTQD_ConfortTqDecSR_Z_Nm/1
  [VTQD_TMSpd_rpm] -> Saturation3/1
  Abs6/1 -> Saturation10/1
  [VTQD_RrRampTq_Nm] -> Abs5/1
  Abs5/1 -> Saturation8/1
  MTQD_ConfortTqDecSR_Z_Nm/1 -> [VTQD_ConfortTqDecSR_Nm]  "VTQD_ConfortTqDecSR_Nm"
  MTQD_ConfortTqIncSR_Z_Nm/1 -> [VTQD_ConfortTqIncSR_Nm]  "VTQD_ConfortTqIncSR_Nm"
  Saturation11/1 -> MTQD_ConfortTqDecSR_Z_Nm/2
  [VTQD_TMSpd_rpm] -> Saturation2/1
  [VTQD_RrRampTq_Nm] -> Abs4/1
  [VTQD_TMSpd_rpm] -> Saturation5/1
  MTQD_NormalTqDecSR_Z_Nm/1 -> [VTQD_NormalTqDecSR_Nm]  "VTQD_NormalTqDecSR_Nm"
  Saturation7/1 -> MTQD_ECOTqDecSR_Z_Nm/2
  Saturation3/1 -> MTQD_NormalTqDecSR_Z_Nm/2
  Abs1/1 -> Saturation1/1
  [VTQD_RrRampTq_Nm] -> Abs/1
  Saturation5/1 -> MTQD_ECOTqIncSR_Z_Nm/2
  MTQD_ECOTqDecSR_Z_Nm/1 -> [VTQD_ECOTqDecSR_Nm]  "VTQD_ECOTqDecSR_Nm"
  Saturation/1 -> MTQD_NormalTqIncSR_Z_Nm/1
  Saturation4/1 -> MTQD_ECOTqIncSR_Z_Nm/1
  Saturation6/1 -> MTQD_ECOTqDecSR_Z_Nm/1
  Saturation8/1 -> MTQD_ConfortTqIncSR_Z_Nm/1
  Saturation1/1 -> MTQD_NormalTqDecSR_Z_Nm/1
  [VTQD_RrRampTq_Nm] -> Abs1/1
  Saturation9/1 -> MTQD_ConfortTqIncSR_Z_Nm/2
  Constant1/1 -> Relational Operator/2
  Relational Operator/1 -> SR_Latch/1
  Detect Decrease/1 -> SR_Latch1/1
  [VTQD_AfterAvailableTqDemRr_Nm] -> Relational Operator/1
  [VTQD_AfterAvailableTqDemRr_Nm] -> Relational Operator1/1
  SR_Latch1/1 -> Counter/1, [VTQD_POSNEGCONVSM_flg]  "VTQD_POSNEGCONVSM_flg"
  OR/1 -> SR_Latch1/2, Counter/2
  KTQD_POSNEGSWSMOTIME_s/1 -> Relational Operator2/2
  Product/1 -> Relational Operator2/1
  Relational Operator2/1 -> Unit Delay/1
  SR_Latch/1 -> Detect Decrease/1
  Unit Delay/1 -> OR/2
  Relational Operator1/1 -> SR_Latch/2
  Counter/1 -> Product/2
  Constant2/1 -> Relational Operator1/2
  [task_time_s] -> Product/1
  Constant4/1 -> Counter/3
  [VTQD_AfterAvailableTqDemRr_Nm] -> Relational Operator3/1
  Constant3/1 -> Relational Operator3/2
  Relational Operator3/1 -> OR/1
  Bus Selector1/1 -> [task_time_s]  "<task_time_s>"
  Bus Selector/2 -> [VTQD_TqSource_enum]  "<VTQD_TqSource_enum>"
  [VTQD_TqSource_enum] -> Ramp Parameter Determination/1(VTQD_TqSource_enum)
  [VTQD_POSNEGCONVSM_flg] -> Ramp Parameter Determination/2(VTQD_POSNEGCONVSM_flg)
  [VTQD_ActDriveMode_enum] -> Ramp Parameter Determination/3(VTQD_ActDriveMode_enum)
  Bus Selector/3 -> [VTQD_ActDriveMode_enum]  "<VTQD_ActDriveMode_enum>"
  [VTQD_NormalTqIncSR_Nm] -> Ramp Parameter Determination/4(VTQD_NormalTqIncSR_Nm)
  [VTQD_NormalTqDecSR_Nm] -> Ramp Parameter Determination/5(VTQD_NormalTqDecSR_Nm)
  [VTQD_ECOTqIncSR_Nm] -> Ramp Parameter Determination/6(VTQD_ECOTqIncSR_Nm)
  [VTQD_ECOTqDecSR_Nm] -> Ramp Parameter Determination/7(VTQD_ECOTqDecSR_Nm)
  [VTQD_ConfortTqIncSR_Nm] -> Ramp Parameter Determination/8(VTQD_ConfortTqIncSR_Nm)
  [VTQD_ConfortTqDecSR_Nm] -> Ramp Parameter Determination/9(VTQD_ConfortTqDecSR_Nm)
  Ramp Parameter Determination/1(VTQD_RampTs_c) -> [VTQD_RampTs_c]
  Ramp Parameter Determination/2(VTQD_RampTqIncSR_Nm) -> [VTQD_RampTqIncSR_Nm]
  Ramp Parameter Determination/3(VTQD_RampTqDecSR_Nm) -> [VTQD_RampTqDecSR_Nm]
  [VTQD_RampTqIncSR_Nm] -> VTQD_RampTqIncSR_Nm/1
  [VTQD_RampTqDecSR_Nm] -> VTQD_RampTqDecSR_Nm/1
  BMain_outputs/1 -> Bus Selector2/1
  Bus Selector2/1 -> [VTQD_RrRampTq_Nm]  "<VTQD_RrRampTq_Nm>"
  Bus Selector2/2 -> [VTQD_AfterAvailableTqDemRr_Nm]  "<VTQD_AfterAvailableTqDemRr_Nm>"
